simulink model "AND1"  (R2014a)
settings: Solver=ode45  StartTime=0.0  StopTime=10.0  RelTol=1e-3
settings Model: Creator=user  LastModifiedBy=user

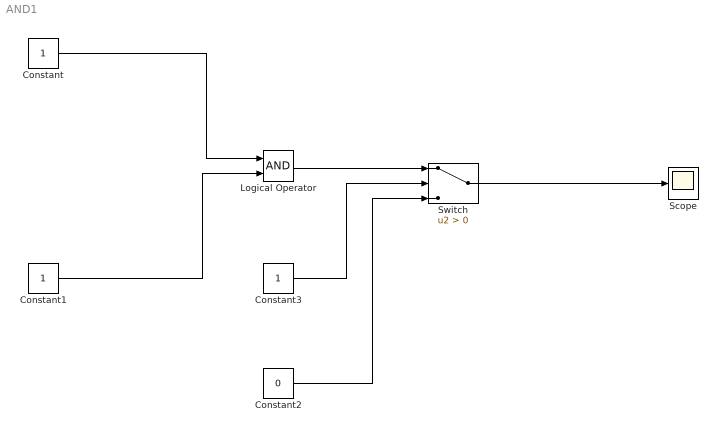
== system AND1 ==
  Constant : Constant
  Constant1 : Constant
  Constant2 : Constant  Value=0
  Constant3 : Constant
  Logical Operator : Logic  AllPortsSameDT=off  OutDataTypeStr=boolean
  Scope : Scope
  Switch : Switch  Criteria=u2 > Threshold
  wires:
  Logical Operator/1 -> Switch/1
  Constant/1 -> Logical Operator/1
  Constant1/1 -> Logical Operator/2
  Switch/1 -> Scope/1
  Constant3/1 -> Switch/2
  Constant2/1 -> Switch/3
